simulink model "test_inputs"  (Simulink 7.6)
settings: Solver=FixedStepDiscrete  StartTime=0.0  StopTime=3  FixedStep=1  RelTol=1e-3
settings Model: Creator=glaurent  LastModifiedBy=guillaume.laurent  ExtModeTrigMode=oneshot  ExtModeArmWhenConnect=off
settings DataIOCC: LimitDataPoints=off
settings OptimizationCC: BlockReduction=off  BooleanDataType=off  InitFltsAndDblsToZero=on
settings DebuggingCC: SaveWithParameterizedLinksMsg=none  SignalResolutionControl=TryResolveAllWithWarning  SolverPrmCheckMsg=none  MultiTaskDSMMsg=warning  MultiTaskCondExecSysMsg=none  StrictBusMsg=None
settings HardwareCC: TargetUnknown=on
settings RTWCC: IncludeERTFirstTime=on
settings GRTTargetCC: ModelReferenceCompliant=off  CompOptLevelCompliant=off  MatFileLogging=off

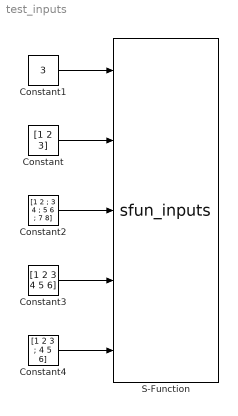
== system test_inputs ==
  Constant : Constant  Value=[1 2 3]
  Constant1 : Constant  Value=3
  Constant2 : Constant  Value=[1 2 ; 3 4 ; 5 6 ; 7 8]
  Constant3 : Constant  Value=[1 2 3 4 5 6]
  Constant4 : Constant  Value=[1 2 3 ; 4 5 6]
  S-Function : S-Function  FunctionName=sfun_inputs  EnableBusSupport=off
  wires:
  Constant1/1 -> S-Function/1
  Constant/1 -> S-Function/2
  Constant2/1 -> S-Function/3
  Constant3/1 -> S-Function/4
  Constant4/1 -> S-Function/5
